simulink model "d2"  (R2013a)
settings: Solver=ode45  StartTime=0.0  StopTime=100.0  FixedStep=0.01  MaxStep=0.005  RelTol=1e-3
undefined symbols (not defined in the file): k2, Tp2
settings Model: Creator=adasdeb  LastModifiedBy=adasdeb
settings DataIOCC: LimitDataPoints=off

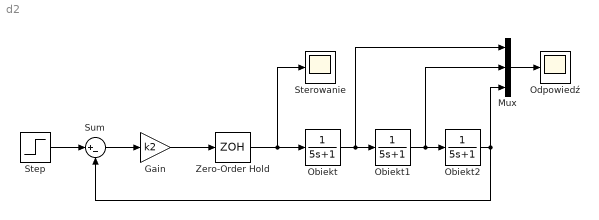
== system d2 ==
  Gain : Gain  Gain=k2
  Mux : Mux  Inputs=3
  Obiekt : TransferFcn  Denominator=[5 1]
  Obiekt1 : TransferFcn  Denominator=[5 1]
  Obiekt2 : TransferFcn  Denominator=[5 1]
  Odpowiedź : Scope
      settings: SaveName=resp3
  Step : Step  SampleTime=0
  Sterowanie : Scope
      settings: SaveName=ster3
  Sum : Sum  Inputs=|+-
  Zero-Order Hold : ZeroOrderHold  SampleTime=Tp2
  wires:
  Sum/1 -> Gain/1
  Gain/1 -> Zero-Order Hold/1
  Zero-Order Hold/1 -> Sterowanie/1, Obiekt/1
  Step/1 -> Sum/1
  Obiekt2/1 -> Mux/3, Sum/2
  Obiekt1/1 -> Obiekt2/1, Mux/2
  Obiekt/1 -> Obiekt1/1, Mux/1
  Mux/1 -> Odpowiedź/1
